simulink model "nsdynamic_YALFA"  (R2021b)
settings: Solver=ode4  StartTime=0.0  StopTime=10.0  RelTol=1e-3
InitFcn:
  | initialization
undefined symbols (not defined in the file or in its folder): dynNS_YALFA, trajectory
settings Model: Creator=AzamaoZ  LastModifiedBy=AzamaoZ

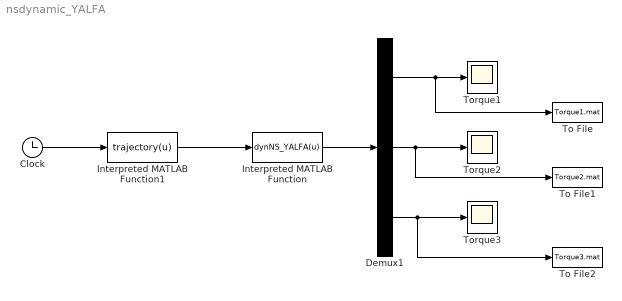
== system nsdynamic_YALFA ==
  Clock : Clock
  Demux1 : Demux  Outputs=3
  Interpreted MATLAB Function : MATLABFcn  MATLABFcn=dynNS_YALFA(u)  OutputDimensions=3
  Interpreted MATLAB Function1 : MATLABFcn  MATLABFcn=trajectory(u)
  To File : ToFile  Filename=Torque1.mat  MatrixName=Torque1  SaveFormat=Timeseries
  To File1 : ToFile  Filename=Torque2.mat  MatrixName=Torque2  SaveFormat=Timeseries
  To File2 : ToFile  Filename=Torque3.mat  MatrixName=Torque3  SaveFormat=Timeseries
  Torque1 : Scope
  Torque2 : Scope
  Torque3 : Scope
  wires:
  Interpreted MATLAB Function/1 -> Demux1/1
  Clock/1 -> Interpreted MATLAB Function1/1
  Demux1/1 -> To File/1, Torque1/1
  Demux1/2 -> Torque2/1, To File1/1
  Demux1/3 -> Torque3/1, To File2/1
  Interpreted MATLAB Function1/1 -> Interpreted MATLAB Function/1
